simulink model "Masa_Resorte_Amortiguador_2"  (R2017a)
settings: Solver=VariableStepAuto  StartTime=0.0  StopTime=80  RelTol=1e-3
InitFcn:
  | m=10
  | b=0.1
  | k=1
  | F=10
  | F1=0
  | F2=0
  | F3=0
  | F4=0
  | F5=0
  | F6=0
  | F7=0
  | w=sqrt(k/m);
  | w1=1
  | w2=1
  | w3=1
  | w4=1
  | w5=1
  | w6=1
  | w7=1
StartFcn:
  | m=2
  | b=0.5
  | k=1
settings Model: Creator=LuisFernando  LastModifiedBy=LuisFernando

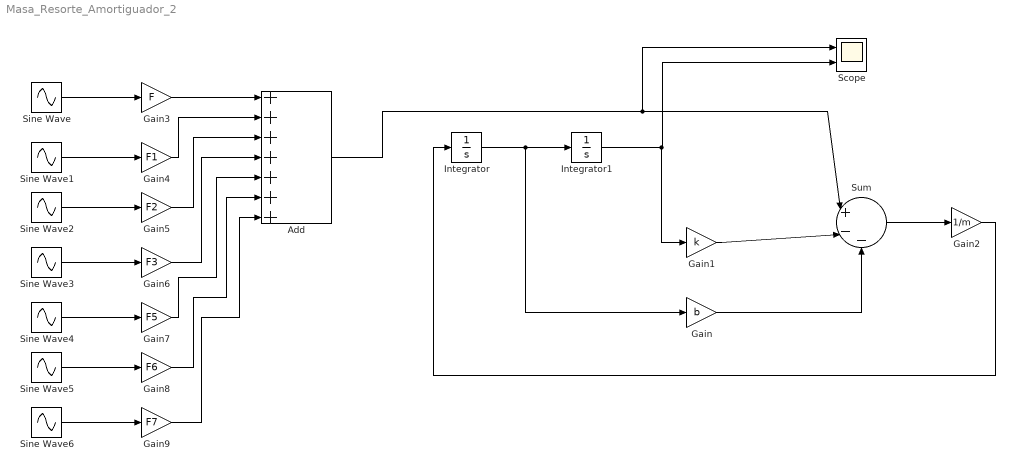
== system Masa_Resorte_Amortiguador_2 ==
  Add : Sum  Inputs=+++++++
  Gain : Gain  Gain=b
  Gain1 : Gain  Gain=k
  Gain2 : Gain  Gain=1/m
  Gain3 : Gain  Gain=F
  Gain4 : Gain  Gain=F1
  Gain5 : Gain  Gain=F2
  Gain6 : Gain  Gain=F3
  Gain7 : Gain  Gain=F5
  Gain8 : Gain  Gain=F6
  Gain9 : Gain  Gain=F7
  Integrator : Integrator  InitialCondition=1
  Integrator1 : Integrator  InitialCondition=2
  Scope : Scope  NumInputPorts=2
  Sine Wave : Sin  Frequency=w  SampleTime=0
  Sine Wave1 : Sin  Frequency=w1  SampleTime=0
  Sine Wave2 : Sin  Frequency=w2  SampleTime=0
  Sine Wave3 : Sin  Frequency=w3  SampleTime=0
  Sine Wave4 : Sin  Frequency=w4  SampleTime=0
  Sine Wave5 : Sin  Frequency=w5  SampleTime=0
  Sine Wave6 : Sin  Frequency=w6  SampleTime=0
  Sum : Sum  Inputs=|+--
  wires:
  Integrator/1 -> Integrator1/1, Gain/1
  Gain1/1 -> Sum/2
  Gain/1 -> Sum/3
  Sum/1 -> Gain2/1
  Gain2/1 -> Integrator/1
  Integrator1/1 -> Gain1/1, Scope/2
  Gain3/1 -> Add/1
  Gain4/1 -> Add/2
  Gain5/1 -> Add/3
  Gain6/1 -> Add/4
  Gain7/1 -> Add/5
  Gain9/1 -> Add/7
  Gain8/1 -> Add/6
  Add/1 -> Scope/1, Sum/1
  Sine Wave/1 -> Gain3/1
  Sine Wave6/1 -> Gain9/1
  Sine Wave5/1 -> Gain8/1
  Sine Wave4/1 -> Gain7/1
  Sine Wave3/1 -> Gain6/1
  Sine Wave2/1 -> Gain5/1
  Sine Wave1/1 -> Gain4/1
